simulink library "MIL_Test"  (Simulink 6.6)
undefined symbols (not defined in the file or in its folder): getdatatypespecs, slcm, StepSize
libraries: simulink x71, MIL_Test x6
(part 2 of 8)

== system MIL_Test/Test Data/Signal comparison/Range - Gap Absolute tolerance Precond ==
  Signal : Inport
  Reference : Inport  Port=2
  Abs : Abs
  Abs1 : Abs
  Absolute Tolerance : Constant  Value=AbsoluteTolerance
  Add : Sum  Inputs=+-  OutScaling=2^-10
  Relational Operator : RelationalOperator  Operator===  LogicOutDataTypeMode=Boolean
  Activate : Outport
  wires:
  Abs1/1 -> Relational Operator/2
  Absolute Tolerance/1 -> Abs1/1
  Reference/1 -> Add/2
  Signal/1 -> Add/1
  Add/1 -> Abs/1
  Abs/1 -> Relational Operator/1
  Relational Operator/1 -> Activate/1

== system MIL_Test/Test Data/Signal comparison/Range - Gap Relative tolerance Precond ==
  Signal : Inport
  Reference : Inport  Port=2
  Abs : Abs
  Abs1 : Abs
  Add : Sum  Inputs=+-  OutScaling=2^-10
  Divide1 : Product  Inputs=**/  OutScaling=2^-10
  Max : Constant  Value=100
  Relational Operator : RelationalOperator  Operator=<=  LogicOutDataTypeMode=Boolean
  Relative Tolerance : Constant
  Activate : Outport
  wires:
  Abs/1 -> Relational Operator/1
  Add/1 -> Abs/1
  Signal/1 -> Add/1
  Reference/1 -> Add/2, Abs1/1
  Divide1/1 -> Relational Operator/2
  Max/1 -> Divide1/3
  Relative Tolerance/1 -> Divide1/2
  Relational Operator/1 -> Activate/1
  Abs1/1 -> Divide1/1

== system MIL_Test/Test Data/Signal comparison/Range - Gap Tolerance range Precond ==
  Signal : Inport
  Lower bound : Inport  Port=2
  Upper bound : Inport  Port=3
  Logical Operator : Logic  AllPortsSameDT=off  OutDataTypeMode=Specify via dialog
  Relational Operator : RelationalOperator  LogicOutDataTypeMode=Boolean
  Relational Operator1 : RelationalOperator  LogicOutDataTypeMode=Boolean
  Activate : Outport
  wires:
  Upper bound/1 -> Relational Operator1/1
  Relational Operator/1 -> Logical Operator/2
  Relational Operator1/1 -> Logical Operator/1
  Signal/1 -> Relational Operator/1, Relational Operator1/2
  Logical Operator/1 -> Activate/1
  Lower bound/1 -> Relational Operator/2

== system MIL_Test/Test Data/Test Data Architecture/<Test data generator> ==
  Test Ctrl Influence : Inport
  Out Bus : Inport  Port=2
  <Requirement name> : Subsystem
  switch <signal1> : MultiPortSwitch  Inputs=1  zeroidx=on
  <signal1> : Outport
  wires:
  Test Ctrl Influence/1 -> switch <signal1>/1
  Out Bus/1 -> <Requirement name>/1(Out Bus)
  switch <signal1>/1 -> <signal1>/1
  <Requirement name>/1(<signal1>) -> switch <signal1>/2

== system MIL_Test/Test Quality/VFs Activation  Coverage/Max to date ==
  Signal : Inport
  Clock : Clock
      settings: Decimation=10
  Memory : Memory  Orientation=left
  MinMax : MinMax  Function=max  Inputs=2
  Switch : Switch  Criteria=u2 > Threshold
  Max : Outport
  wires:
  Memory/1 -> Switch/1
  Clock/1 -> Switch/2
  Switch/1 -> MinMax/1
  Signal/1 -> Switch/3, MinMax/2
  MinMax/1 -> Memory/1, Max/1

== system MIL_Test/Test Quality/VFs Activation  Coverage/Max to date1 ==
  Signal : Inport
  Clock : Clock
      settings: Decimation=10
  Memory : Memory  Orientation=left
  MinMax : MinMax  Function=max  Inputs=2
  Switch : Switch  Criteria=u2 > Threshold
  Max : Outport
  wires:
  Memory/1 -> Switch/1
  Clock/1 -> Switch/2
  Switch/1 -> MinMax/1
  Signal/1 -> Switch/3, MinMax/2
  MinMax/1 -> Memory/1, Max/1

== system MIL_Test/Validation Function/Feature extraction/Complete step detection ==
  Step : Inport
  Step response : Inport  Port=2
  Step detection : Subsystem  mask{MT=10, RT=0.001}
      mask prompts: MT "Minimal time for signals to be constant before a step"; RT "Relative tolerance for constant detection in %"
      mask CallbackString:
      | if (str2double(get_param(gcb,'MT')) < 0)
      |     error(['Minimal time specified (' get_param(gcb,'MT') ') negative. Please give a non-negative value.']);
      | else
      |     set_param([gcb '/Active if signals constant for some specified time/Min Time'],'Value',get_param(gcb,'MT'));
      | end|if or( (str2double(get_param(gcb,'RT')) < 0), (str2double(get_param(gcb,'RT')) > 100))
      |     error(['Relative tolerance value (' get_param(gcb,'RT') ') out of range. Please give a value between 0 and 100.']);
      | else
      |     set_param([gcb '/Active if signals constant for some specified time/Time since signal constant/Detect constant/Relative tolerance/Relative Tolerance'],'Value',get_param(gcb,'RT'));
      |     set_param([gcb '/Active if signals constant for some specified time/Time since signal constant/Detect constant'],'RT',get_param(gcb,'RT'));
      |     set_param([gcb '/Active if signals constant for some specified time/Time since signal constant'],'RT',get_param(gcb,'RT'));
      |     set_param([gcb '/Active if signals constant for some specified time/Time since signal constant1/Detect constant/Relative tolerance/Relative Tolerance'],'Value',get_param(gcb,'RT'));
      |     set_param([gcb '/Active if signals constant for some specified time/Time since signal constant1/Detect constant'],'RT',get_param(gcb,'RT'));
      |     set_param([gcb '/Active if signals constant for some specified time/Time since signal constant1'],'RT',get_param(gcb,'RT'));
      | end
  Step detection reset : Subsystem  mask{MT=10, RT=0.0001, MSS=10}
      mask prompts: MT "Minimal time for signals to be constant before a step"; RT "Relative tolerance for constant detection in %"; MSS "Minimal step size for step detection"
      mask CallbackString:
      | if (str2double(get_param(gcb,'MT')) < 0)
      |     error(['Minimal time specified (' get_param(gcb,'MT') ') negative. Please give a non-negative value.']);
      | else
      |     set_param([gcb '/Active if signals constant for some specified time/Min Time'],'Value',get_param(gcb,'MT'));
      | end|if or( (str2double(get_param(gcb,'RT')) < 0), (str2double(get_param(gcb,'RT')) > 100))
      |     error(['Relative tolerance value (' get_param(gcb,'RT') ') out of range. Please give a value between 0 and 100.']);
      | else
      |     set_param([gcb '/Active if signals constant for some specified time/Time since signal constant/Detect constant/Relative tolerance/Relative Tolerance'],'Value',get_param(gcb,'RT'));
      |     set_param([gcb '/Active if signals constant for some specified time/Time since signal constant/Detect constant'],'RT',get_param(gcb,'RT'));
      |     set_param([gcb '/Active if signals constant for some specified time/Time since signal constant'],'RT',get_param(gcb,'RT'));
      |     set_param([gcb '/Active if signals constant for some specified time/Time since signal constant1/Detect constant/Relative tolerance/Relative Tolerance'],'Value',get_param(gcb,'RT'));
      |     set_param([gcb '/Active if signals constant for some specified time/Time since signal constant1/Detect constant'],'RT',get_param(gcb,'RT'));
      |     set_param([gcb '/Active if signals constant for some specified time/Time since signal constant1'],'RT',get_param(gcb,'RT'));
      | end|if (str2double(get_param(gcb,'MSS')) < 0)
      |     error(['Minimal step size specified (' get_param(gcb,'MSS') ') negative. Please give a non-negative value.']);
      | else
      |     set_param([gcb '/Step detection/Min step size'],'Value',get_param(gcb,'MSS'));
      |     set_param([gcb '/Step detection'],'StepSize',get_param(gcb,'MSS'));
      | 
      | end
  R : Outport
  T : Outport  Port=2
  Complete step : Outport  Port=3
  wires:
  Step detection/1(End of complete step) -> T/1, Complete step/1
  Step detection reset/1(R) -> R/1, Step detection/1(R)
  Step response/1 -> Step detection reset/2(Step response), Step detection/3(Step response)
  Step/1 -> Step detection reset/1(Step), Step detection/2(Step)

== system MIL_Test/Validation Function/Feature extraction/Detect constant ==
  Signal : Inport
  Clock : Clock
      settings: Decimation=10
  Constant1 : Constant  Value=0  OutDataTypeMode=boolean
  Memory : Memory
  Relative tolerance : Subsystem
  Switch : Switch  Criteria=u2 > Threshold
  Constant : Outport
  wires:
  Switch/1 -> Constant/1
  Relative tolerance/1(sig == ref) -> Switch/1
  Clock/1 -> Switch/2
  Constant1/1 -> Switch/3
  Memory/1 -> Relative tolerance/2(ref)
  Signal/1 -> Relative tolerance/1(sig), Memory/1

== system MIL_Test/Validation Function/Feature extraction/Detect decrease ==
  Signal : Inport
  Clock : Clock
      settings: Decimation=10
  Memory : Memory
  Relational Operator : RelationalOperator  Operator=<  LogicOutDataTypeMode=Specify via dialog
  Switch : Switch  Criteria=u2 > Threshold
  Decrease : Outport
  wires:
  Signal/1 -> Relational Operator/1, Memory/1, Switch/3
  Relational Operator/1 -> Decrease/1
  Clock/1 -> Switch/2
  Memory/1 -> Switch/1
  Switch/1 -> Relational Operator/2

== system MIL_Test/Validation Function/Feature extraction/Detect increase ==
  Signal : Inport
  Clock : Clock
      settings: Decimation=10
  Memory : Memory
  Relational Operator : RelationalOperator  Operator=>  LogicOutDataTypeMode=Specify via dialog
  Switch : Switch  Criteria=u2 > Threshold
  Increase : Outport
  wires:
  Switch/1 -> Relational Operator/2
  Memory/1 -> Switch/1
  Clock/1 -> Switch/2
  Relational Operator/1 -> Increase/1
  Signal/1 -> Switch/3, Memory/1, Relational Operator/1

== system MIL_Test/Validation Function/Feature extraction/Linear relation ==
  y : Inport
  u : Inport  Port=2
  Product : Product  RndMeth=Zero
  Relative tolerance : Subsystem
  c : Constant  Value=5
  y == c u : Outport
  wires:
  Relative tolerance/1(sig == ref) -> y == c u/1
  c/1 -> Product/2
  u/1 -> Product/1
  Product/1 -> Relative tolerance/2(ref)
  y/1 -> Relative tolerance/1(sig)

== system MIL_Test/Validation Function/Feature extraction/Local maximum ==
  Signal : Inport
  Clock : Clock
      settings: Decimation=10
  Clock1 : Clock
      settings: Decimation=10
  Logical Operator : Logic  AllPortsSameDT=off  OutDataTypeMode=Boolean
  Memory : Memory
  Memory1 : Memory
  Relational Operator : RelationalOperator  Operator=<  LogicOutDataTypeMode=Boolean
  Relational Operator1 : RelationalOperator  Operator=>  LogicOutDataTypeMode=Boolean
  Switch : Switch  Criteria=u2 > Threshold
  Switch1 : Switch  Criteria=u2 > Threshold
  Maximum : Outport
  wires:
  Switch1/1 -> Relational Operator1/2
  Memory1/1 -> Switch1/1
  Clock1/1 -> Switch1/2
  Switch/1 -> Relational Operator1/1, Switch1/3, Memory1/1, Relational Operator/2
  Memory/1 -> Switch/1
  Clock/1 -> Switch/2
  Relational Operator/1 -> Logical Operator/1
  Relational Operator1/1 -> Logical Operator/2
  Logical Operator/1 -> Maximum/1
  Signal/1 -> Switch/3, Memory/1, Relational Operator/1

== system MIL_Test/Validation Function/Feature extraction/Min to date ==
  Signal : Inport
  Clock : Clock
      settings: Decimation=10
  Memory : Memory  Orientation=left
  MinMax : MinMax  Inputs=2
  Switch : Switch  Criteria=u2 > Threshold
  Min : Outport
  wires:
  Memory/1 -> Switch/1
  Clock/1 -> Switch/2
  Switch/1 -> MinMax/1
  Signal/1 -> Switch/3, MinMax/2
  MinMax/1 -> Memory/1, Min/1

== system MIL_Test/Validation Function/Feature extraction/Moving average ==
  Signal : Inport
  Add : Sum  OutScaling=2^-10
  Clock : Clock
      settings: Decimation=10
  Constant : Constant  Value=2
  Divide : Product  Inputs=*/  OutScaling=2^-10
  Memory : Memory
  Switch : Switch  Criteria=u2 > Threshold
  MA : Outport
  wires:
  Switch/1 -> Add/2
  Memory/1 -> Switch/1
  Clock/1 -> Switch/2
  Signal/1 -> Add/1, Switch/3, Memory/1
  Add/1 -> Divide/1
  Constant/1 -> Divide/2
  Divide/1 -> MA/1

== system MIL_Test/Validation Function/Feature extraction/Peak detection ==
  Signal : Inport
  Abs : Abs
  Abs1 : Abs
  Add : Sum  Inputs=+-  OutScaling=2^-10
  Add1 : Sum  Inputs=+-  OutScaling=2^-10
  Clock : Clock
      settings: Decimation=10
  Clock1 : Clock
      settings: Decimation=10
  Compare To Zero : simulink/Logic and Bit Operations/Compare To Zero  SystemSampleTime=-1  relop=<=  LogicOutDataTypeMode=boolean  ZeroCross=off
  Logical Operator : Logic  Inputs=3  AllPortsSameDT=off  OutDataTypeMode=Boolean
  Memory : Memory
  Memory1 : Memory
  Product : Product  RndMeth=Zero
  Relational Operator : RelationalOperator  Operator=<=  LogicOutDataTypeMode=Boolean
  Relational Operator1 : RelationalOperator  LogicOutDataTypeMode=Boolean
  Sensibility1 : Constant  Value=0.198
  Sensibility2 : Constant  Value=0.198
  Switch : Switch  Criteria=u2 > Threshold
  Switch1 : Switch  Criteria=u2 > Threshold
  Peak : Outport
  wires:
  Sensibility2/1 -> Relational Operator1/2
  Abs1/1 -> Relational Operator1/1
  Sensibility1/1 -> Relational Operator/1
  Abs/1 -> Relational Operator/2
  Product/1 -> Compare To Zero/1
  Compare To Zero/1 -> Logical Operator/2
  Relational Operator1/1 -> Logical Operator/3
  Relational Operator/1 -> Logical Operator/1
  Add1/1 -> Product/2, Abs1/1
  Signal/1 -> Memory/1, Switch/3, Add/1
  Logical Operator/1 -> Peak/1
  Clock/1 -> Switch/2
  Memory/1 -> Switch/1
  Switch/1 -> Add1/1, Add/2, Memory1/1, Switch1/3
  Clock1/1 -> Switch1/2
  Memory1/1 -> Switch1/1
  Switch1/1 -> Add1/2
  Add/1 -> Product/1, Abs/1

== system MIL_Test/Validation Function/Feature extraction/Signal value @ maximum ==
  Signal : Inport
  Local maximum : Subsystem  TreatAsAtomicUnit=on
  Trigger : Outport
  Feature : Outport  Port=2
  wires:
  Local maximum/1(Maximum) -> Trigger/1
  Signal/1 -> Local maximum/1(Signal), Feature/1

== system MIL_Test/Validation Function/Feature extraction/Step detection ==
  Signal : Inport
  Abs : Abs
  Add : Sum  Inputs=+-  OutScaling=2^-10
  Clock : Clock
      settings: Decimation=10
  Memory : Memory
  Min step size : Constant
  Relational Operator : RelationalOperator  LogicOutDataTypeMode=Boolean
  Switch : Switch  Criteria=u2 > Threshold
  Step : Outport
  wires:
  Switch/1 -> Add/2
  Memory/1 -> Switch/1
  Clock/1 -> Switch/2
  Signal/1 -> Add/1, Switch/3, Memory/1
  Abs/1 -> Relational Operator/1
  Min step size/1 -> Relational Operator/2
  Relational Operator/1 -> Step/1
  Add/1 -> Abs/1

== system MIL_Test/Validation Function/Feature extraction/Step response characteristics ==
  Step : Inport
  Step response : Inport  Port=2
  Step response characteristics extraction : Subsystem  mask(Step response feature extraction){gain=0.8333, lowerLim=10, upperLim=90, MOma=ones(1,10), RelTol=0.1, MinTime=1, Range=5, sseW=ones(1,10)}
      mask prompts: gain "System's static gain"; lowerLim "Rise time interval lower limit (in set point %)"; upperLim "Rise time interval upper limit (in set point %)"; MOma "Maximum overshoot moving average weights"; RelTol "Maximum overshoot - Detect constant if no overshoot - Relative Tolerance"; MinTime "Maximum overshoot - Detect constant if no overshoot - Minimum constant time"; Range "Settling time range (in set point %)"; sseW "Steady state error - moving average weights"
      mask help: Extracts four step response feature characteristics. Extraction parameters are shown below.
      mask CallbackString:
      | set_param([gcb '/Static Gain'],'Value',get_param(gcb,'gain'));|set_param([gcb '/Extract rise time/lowerLim'],'Value',get_param(gcb,'lowerLim'));|set_param([gcb '/Extract rise time/upperLim'],'Value',get_param(gcb,'upperLim'));|set_param([gcb '/Extract maximum overshoot/Step response moving average and initial conditions before step/Weighted Moving Average'],'mgainval',get_param(gcb,'MOma'));
      | set_param([gcb '/Extract maximum overshoot/Step response moving average and initial conditions before step/Weighted Moving Average1'],'mgainval',get_param(gcb,'MOma'));|set_param([gcb '/Extract maximum overshoot/Active if signals constant for some specified time/Time since signal constant'],'RT',get_param(gcb,'RelTol'));
      | set_param([gcb '/Extract maximum overshoot/Active if signals constant for some specified time/Time since signal constant1'],'RT',get_param(gcb,'RelTol'));|set_param([gcb '/Extract maximum overshoot/Active if signals constant for some specified time/Min Time'],'Value',get_param(gcb,'MinTime'));|set_param([gcb '/Extract settling time/Set point percent'],'Value',get_param(gcb,'Range'));|set_param([gcb '/Extract steady state error/Weighted Moving Average'],'mgainval',get_param(gcb,'sseW'));
  Step response reset : Subsystem  mask{MT=1, RT=0.0001, MSS=1}
      mask prompts: MT "Minimal time for signals to be constant before a step"; RT "Relative tolerance for constant detection in %"; MSS "Minimal step size for step detection"
      mask CallbackString:
      | if (str2double(get_param(gcb,'MT')) < 0)
      |     error(['Minimal time specified (' get_param(gcb,'MT') ') negative. Please give a non-negative value.']);
      | else
      |     set_param([gcb '/Active if signals constant for some specified time/Min Time'],'Value',get_param(gcb,'MT'));
      | end|if or( (str2double(get_param(gcb,'RT')) < 0), (str2double(get_param(gcb,'RT')) > 100))
      |     error(['Relative tolerance value (' get_param(gcb,'RT') ') out of range. Please give a value between 0 and 100.']);
      | else
      |     set_param([gcb '/Active if signals constant for some specified time/Time since signal constant/Detect constant/Relative tolerance/Relative Tolerance'],'Value',get_param(gcb,'RT'));
      |     set_param([gcb '/Active if signals constant for some specified time/Time since signal constant/Detect constant'],'RT',get_param(gcb,'RT'));
      |     set_param([gcb '/Active if signals constant for some specified time/Time since signal constant'],'RT',get_param(gcb,'RT'));
      |     set_param([gcb '/Active if signals constant for some specified time/Time since signal constant1/Detect constant/Relative tolerance/Relative Tolerance'],'Value',get_param(gcb,'RT'));
      |     set_param([gcb '/Active if signals constant for some specified time/Time since signal constant1/Detect constant'],'RT',get_param(gcb,'RT'));
      |     set_param([gcb '/Active if signals constant for some specified time/Time since signal constant1'],'RT',get_param(gcb,'RT'));
      | end|if (str2double(get_param(gcb,'MSS')) < 0)
      |     error(['Minimal step size specified (' get_param(gcb,'MSS') ') negative. Please give a non-negative value.']);
      | else
      |     set_param([gcb '/Step detection/Min step size'],'Value',get_param(gcb,'MSS'));
      |     set_param([gcb '/Step detection'],'StepSize',get_param(gcb,'MSS'));
      | 
      | end
  Step response trigger : Subsystem  mask(Step response trigger extraction){MinTime=1, RelTol=0.5, MAXsse=0.5}
      mask prompts: MinTime "Detect constant signals - Minimum constant time"; RelTol "Detect constant signals - Relative Tolerance"; MAXsse "Maximum steady state error for triggering"
      mask help: This block extracts the trigger signals for the four step response characteristics.
      mask CallbackString:
      | set_param([gcb '/Active if signals constant for some specified time/Min Time'],'Value',get_param(gcb,'MinTime'));|set_param([gcb '/Active if signals constant for some specified time/Time since signal constant'],'RT',get_param(gcb,'RelTol'));
      | set_param([gcb '/Active if signals constant for some specified time/Time since signal constant1'],'RT',get_param(gcb,'RelTol'));|set_param([gcb '/Compare To Constant'],'const',get_param(gcb,'MAXsse'));
  R : Outport
  Rise time T : Outport  Port=2  DataType=double
  Overshoot T : Outport  Port=3  DataType=double
  Settling time T : Outport  Port=4  DataType=double
  Steady state error T : Outport  Port=5  DataType=double
  Rise time : Outport  Port=6
  Maximum Overshoot : Outport  Port=7
  Settling time : Outport  Port=8  DataType=double
  Steady state error : Outport  Port=9  DataType=double
  wires:
  Step response trigger/4(Steady state error T) -> Steady state error T/1
  Step response trigger/3(Settling time T) -> Settling time T/1
  Step response trigger/2(Overshoot T) -> Overshoot T/1
  Step response trigger/1(Rise time T) -> Rise time T/1
  Step response characteristics extraction/2(Maximum overshoot) -> Maximum Overshoot/1
  Step response characteristics extraction/3(Settling time) -> Settling time/1
  Step response characteristics extraction/1(Rise time) -> Rise time/1
  Step response/1 -> Step response trigger/2(Step response), Step response characteristics extraction/3(Step response), Step response reset/2(Step response)
  Step/1 -> Step response characteristics extraction/2(Step), Step response reset/1(Step)
  Step response characteristics extraction/4(Steady state error) -> Steady state error/1, Step response trigger/1(Steady state error)
  Step response reset/1(R) -> Step response characteristics extraction/1(R), R/1

== system MIL_Test/Validation Function/Feature extraction/Time @ sig = x ==
  Signal : Inport
  Clock : Clock
      settings: Decimation=10
  Relative tolerance : Subsystem
  Trigger Value : Constant  Value=5
  Trigger : Outport
  Feature : Outport  Port=2
  wires:
  Clock/1 -> Feature/1
  Trigger Value/1 -> Relative tolerance/2(ref)
  Signal/1 -> Relative tolerance/1(sig)
  Relative tolerance/1(sig == ref) -> Trigger/1

== system MIL_Test/Validation Function/Feature extraction/Time since signal constant ==
  Signal : Inport
  Clock : Clock
      settings: Decimation=10
  Detect constant : Subsystem  TreatAsAtomicUnit=on  mask(Feature extraction block){RT=1}
      mask prompts: RT "Relative tolerance in %"
      mask help: Detect if the signal value is constant (using the last two signal values) allowing for a user-defined relative deviation
      mask CallbackString:
      | if or( (str2double(get_param(gcb,'RT')) < 0), (str2double(get_param(gcb,'RT')) > 100))
      |     error(['Relative tolerance value (' get_param(gcb,'RT') ') out of range. Please give a value between 0 and 100.']);
      | else
      |     set_param([gcb '/Relative tolerance/Relative Tolerance'],'Value',get_param(gcb,'RT'));
      | end
  Logical Operator : Logic  Operator=NAND  AllPortsSameDT=off  OutDataTypeMode=Boolean
  Logical Operator1 : Logic  Operator=NOT  AllPortsSameDT=off  OutDataTypeMode=Boolean
  Memory : Memory  Orientation=left
  Memory1 : Memory
  Subtract : Sum  Inputs=-+  OutScaling=2^-10
  Switch : Switch  Criteria=u2 > Threshold
  Trigger : Outport
  Feature : Outport  Port=2
  wires:
  Logical Operator/1 -> Switch/2
  Logical Operator1/1 -> Logical Operator/2
  Memory1/1 -> Logical Operator1/1
  Memory/1 -> Switch/1
  Switch/1 -> Memory/1, Subtract/1
  Clock/1 -> Switch/3, Subtract/2
  Subtract/1 -> Feature/1
  Detect constant/1(Constant) -> Memory1/1, Logical Operator/1, Trigger/1
  Signal/1 -> Detect constant/1(Signal)

== system MIL_Test/Validation Function/Signal comparison/Bound Ass ==
  Signal : Inport
  Reference : Inport  Port=2
  Bus Creator : BusCreator  Inputs=5
  Data Type Conversion{,1..3} (4 alike) : DataTypeConversion
  Delay : Constant  Value=0
  LOWER : Constant  Value=Lower  OutDataTypeMode=int8
  No Limit : Constant  Value=Inf
  No limit : Constant  Value=-Inf
  Relational Operator : RelationalOperator  Operator=<=  LogicOutDataTypeMode=Boolean  LogicDataType=double
  Switch 2 : Switch  Criteria=u2 ~= 0
  Switch 3 : Switch  Criteria=u2 ~= 0
  UPPER : Constant  Value=Upper  OutDataTypeMode=int8
  V : Outport  InitialOutput=[2]
  wires:
  Relational Operator/1 -> Data Type Conversion/1
  Data Type Conversion3/1 -> Bus Creator/4  "Actual data"
  Data Type Conversion2/1 -> Bus Creator/3  "Expected upper limit"
  Data Type Conversion1/1 -> Bus Creator/2  "Expected lower limit"
  Data Type Conversion/1 -> Bus Creator/1  "Local verdict"
  Bus Creator/1 -> V/1
  Reference/1 -> Relational Operator/2, Switch 2/3, Switch 3/3
  Signal/1 -> Data Type Conversion3/1, Relational Operator/1
  UPPER/1 -> Switch 3/2
  No Limit/1 -> Switch 3/1
  LOWER/1 -> Switch 2/2
  No limit/1 -> Switch 2/1
  Switch 2/1 -> Data Type Conversion1/1
  Switch 3/1 -> Data Type Conversion2/1
  Delay/1 -> Bus Creator/5  "Delay"

== system MIL_Test/Validation Function/Signal comparison/Bound Precond ==
  Signal : Inport
  Reference : Inport  Port=2
  RelOp : RelationalOperator  LogicOutDataTypeMode=Specify via dialog
  Activate : Outport
  wires:
  Signal/1 -> RelOp/1
  RelOp/1 -> Activate/1
  Reference/1 -> RelOp/2

== system MIL_Test/Validation Function/Signal comparison/Range - Gap Absolute tolerance Ass ==
  Signal : Inport
  Reference : Inport  Port=2
  Abs : Abs
  Abs1 : Abs
  Absolute Tolerance : Constant  Value=AbsoluteTolerance
  Add : Sum  Inputs=+-  OutScaling=2^-10
  Add1 : Sum  Inputs=+-  OutScaling=2^-10
  Add2 : Sum  OutScaling=2^-10
  Bus Creator : BusCreator  Inputs=5
  Data Type Conversion{,1..3} (4 alike) : DataTypeConversion
  Delay : Constant  Value=0
  Relational Operator : RelationalOperator  Operator===  LogicOutDataTypeMode=Boolean
  V : Outport  InitialOutput=[2]
  wires:
  Abs1/1 -> Relational Operator/2, Add2/2, Add1/2
  Absolute Tolerance/1 -> Abs1/1
  Reference/1 -> Add/2, Add2/1, Add1/1
  Signal/1 -> Add/1, Data Type Conversion3/1
  Add/1 -> Abs/1
  Abs/1 -> Relational Operator/1
  Relational Operator/1 -> Data Type Conversion/1
  Delay/1 -> Bus Creator/5  "Delay"
  Add2/1 -> Data Type Conversion2/1
  Add1/1 -> Data Type Conversion1/1
  Bus Creator/1 -> V/1
  Data Type Conversion/1 -> Bus Creator/1  "Local verdict"
  Data Type Conversion1/1 -> Bus Creator/2  "Expected lower limit"
  Data Type Conversion2/1 -> Bus Creator/3  "Expected upper limit"
  Data Type Conversion3/1 -> Bus Creator/4  "Actual data"

== system MIL_Test/Validation Function/Signal comparison/Range - Gap Absolute tolerance Precond ==
  Signal : Inport
  Reference : Inport  Port=2
  Abs : Abs
  Abs1 : Abs
  Absolute Tolerance : Constant  Value=AbsoluteTolerance
  Add : Sum  Inputs=+-  OutScaling=2^-10
  Relational Operator : RelationalOperator  Operator===  LogicOutDataTypeMode=Boolean
  Activate : Outport
  wires:
  Relational Operator/1 -> Activate/1
  Abs/1 -> Relational Operator/1
  Add/1 -> Abs/1
  Signal/1 -> Add/1
  Reference/1 -> Add/2
  Absolute Tolerance/1 -> Abs1/1
  Abs1/1 -> Relational Operator/2

== system MIL_Test/Validation Function/Signal comparison/Range - Gap Relative tolerance Ass ==
  Signal : Inport
  Reference : Inport  Port=2
  Abs : Abs
  Abs1 : Abs
  Add : Sum  Inputs=+-  OutScaling=2^-10
  Add1 : Sum  Inputs=+-  OutScaling=2^-10
  Add2 : Sum  OutScaling=2^-10
  Bus Creator : BusCreator  Inputs=5
  Data Type Conversion{,1..3} (4 alike) : DataTypeConversion
  Delay : Constant  Value=0
  Divide1 : Product  Inputs=**/  OutScaling=2^-10
  Max : Constant  Value=100
  Relational Operator : RelationalOperator  Operator=<=  LogicOutDataTypeMode=Boolean
  Relative Tolerance : Constant
  V : Outport  InitialOutput=[2]
  wires:
  Abs/1 -> Relational Operator/1
  Add/1 -> Abs/1
  Signal/1 -> Add/1, Data Type Conversion3/1
  Reference/1 -> Add/2, Abs1/1, Add2/2, Add1/1
  Divide1/1 -> Relational Operator/2, Add1/2, Add2/1
  Max/1 -> Divide1/3
  Relative Tolerance/1 -> Divide1/2
  Relational Operator/1 -> Data Type Conversion/1
  Abs1/1 -> Divide1/1
  Delay/1 -> Bus Creator/5  "Delay"
  Add2/1 -> Data Type Conversion2/1
  Add1/1 -> Data Type Conversion1/1
  Bus Creator/1 -> V/1
  Data Type Conversion/1 -> Bus Creator/1  "Local verdict"
  Data Type Conversion1/1 -> Bus Creator/2  "Expected lower limit"
  Data Type Conversion2/1 -> Bus Creator/3  "Expected upper limit"
  Data Type Conversion3/1 -> Bus Creator/4  "Actual data"

== system MIL_Test/Validation Function/Signal comparison/Range - Gap Relative tolerance Precond ==
  Signal : Inport
  Reference : Inport  Port=2
  Abs : Abs
  Abs1 : Abs
  Add : Sum  Inputs=+-  OutScaling=2^-10
  Divide1 : Product  Inputs=**/  OutScaling=2^-10
  Max : Constant  Value=100
  Relational Operator : RelationalOperator  Operator=<=  LogicOutDataTypeMode=Boolean
  Relative Tolerance : Constant
  Activate : Outport
  wires:
  Abs1/1 -> Divide1/1
  Relational Operator/1 -> Activate/1
  Relative Tolerance/1 -> Divide1/2
  Max/1 -> Divide1/3
  Divide1/1 -> Relational Operator/2
  Reference/1 -> Abs1/1, Add/2
  Signal/1 -> Add/1
  Add/1 -> Abs/1
  Abs/1 -> Relational Operator/1

== system MIL_Test/Validation Function/Signal comparison/Range - Gap Tolerance range Ass ==
  Signal : Inport
  Lower bound : Inport  Port=2
  Upper bound : Inport  Port=3
  Bus Creator : BusCreator  Inputs=5
  Data Type Conversion{,1..3} (4 alike) : DataTypeConversion
  Delay : Constant  Value=0
  Logical Operator : Logic  AllPortsSameDT=off  OutDataTypeMode=Specify via dialog
  Relational Operator : RelationalOperator  LogicOutDataTypeMode=Boolean
  Relational Operator1 : RelationalOperator  LogicOutDataTypeMode=Boolean
  V : Outport  InitialOutput=[2]
  wires:
  Upper bound/1 -> Relational Operator1/1, Data Type Conversion2/1
  Relational Operator/1 -> Logical Operator/2
  Relational Operator1/1 -> Logical Operator/1
  Signal/1 -> Relational Operator/1, Relational Operator1/2, Data Type Conversion3/1
  Logical Operator/1 -> Data Type Conversion/1
  Lower bound/1 -> Relational Operator/2, Data Type Conversion1/1
  Delay/1 -> Bus Creator/5  "Delay"
  Bus Creator/1 -> V/1
  Data Type Conversion/1 -> Bus Creator/1  "Local verdict"
  Data Type Conversion1/1 -> Bus Creator/2  "Expected lower limit"
  Data Type Conversion2/1 -> Bus Creator/3  "Expected upper limit"
  Data Type Conversion3/1 -> Bus Creator/4  "Actual data"

== system MIL_Test/Validation Function/Signal comparison/Range - Gap Tolerance range Precond ==
  Signal : Inport
  Lower bound : Inport  Port=2
  Upper bound : Inport  Port=3
  Logical Operator : Logic  AllPortsSameDT=off  OutDataTypeMode=Specify via dialog
  Relational Operator : RelationalOperator  LogicOutDataTypeMode=Boolean
  Relational Operator1 : RelationalOperator  LogicOutDataTypeMode=Boolean
  Activate : Outport
  wires:
  Lower bound/1 -> Relational Operator/2
  Logical Operator/1 -> Activate/1
  Signal/1 -> Relational Operator1/2, Relational Operator/1
  Relational Operator1/1 -> Logical Operator/1
  Relational Operator/1 -> Logical Operator/2
  Upper bound/1 -> Relational Operator1/1

== system MIL_Test/Validation Function/TODO/<system name> ==
  InOut Bus : Inport
  <Requirement name> : Subsystem  Description=Requirement template. Create a new requirement from this template.
  Bus Creator : BusCreator  Inputs=1
  Signal Conversion : SignalConversion  ConversionOutput=Bus copy
  Terminator : Terminator
  wires:
  InOut Bus/1 -> Signal Conversion/1
  Bus Creator/1 -> Terminator/1
  <Requirement name>/1(Test Info) -> Bus Creator/1
  Signal Conversion/1 -> <Requirement name>/1(InOut Bus)

== system MIL_Test/Validation Function/TODO/Assertions ==
  Activate : Inport
  InOut Bus : Inport  Port=2
  Fault info : Subsystem  TreatAsAtomicUnit=on  mask{Ass=[65   99   99   80  101  100   97  108   32   61   61   32   49], Pre=[73  110   79  117  116   10   66  117  115], Req=[83   82   45   80   73   45   48   49   46   51   10   65   99   99  101  108  101  114   97  116  105  111  110   10   80  101  100   97  108   32  114  101   99  111  103  110  105  116  105  111  110]}
      mask prompts: Req "Mask Parameter 3:"
      mask init:
      | set_param(gcb, ...
      |           'Ass', ...
      |           ['[' num2str(uint8(get_param(get_param(gcb,'Parent'),'Name'))) ']']);
      | LinesToAss = getfield(get_param(get_param(get_param(gcb,'Parent'),'handle'),'LineHandles'),'Inport');
      | LinePreToAss = LinesToAss(1);
      | set_param(gcb, ...
      |           'Pre', ...
      |           ['[' num2str(uint8(get_param(get_param(LinePreToAss,'SrcBlockHandle'),'Name'))) ']']); 
      | set_param(gcb, ...
      |           'Req', ...
      |           ['[' num2str(uint8(get_param(get_param(get_param(get_param(gcb,'Parent'),'handle'),'Parent'),'Name'))) ']']);
      | clear LinesToAss LinePreToAss;
  Signal comparison : Subsystem
  VF info : Outport

== system MIL_Test/Validation Function/TODO/Model Info ==
  EmptySubsystem : Subsystem

== system MIL_Test/Validation Function/TODO/Preconditions ==
  Signal comparison : Subsystem

== system MIL_Test/Validation Function/TODO/TD determinate (TD D) ==
  Signal : Inport
  Trigger : Outport
  Feature : Outport  Port=2

== system MIL_Test/Validation Function/TODO/TD immediate (TD I) ==
  Signal : Inport
  Trigger : Outport
  Feature : Outport  Port=2

== system MIL_Test/Validation Function/TODO/TD indeterminate ==
  Signal : Inport
  R : Outport
  T : Outport  Port=2
  Feature : Outport  Port=3

== system MIL_Test/Validation Function/TODO/TD indeterminate, limited (TD IL) ==
  Signal : Inport
  R : Outport
  T : Outport  Port=2
  Feature : Outport  Port=3

== system MIL_Test/Validation Function/TODO/TI determinate (TI D) ==
  Signal : Inport
  Feature : Outport

== system MIL_Test/Validation Function/TODO/TI immediate (TI I) ==
  Signal : Inport
  Feature : Outport

== system MIL_Test/Validation Function/TODO/Validation FunctionsTemplate ==
  InOut Bus : Inport
  Arbitration : Subsystem
  Bus Creator : BusCreator  Inputs=2
  Bus Creator4 : BusCreator  Inputs=2
  Bus Selector : BusSelector  OutputSignals=signal1.signal1
  Datatype conversion : Subsystem  TreatAsAtomicUnit=on
  Requirement : Subsystem  mask{No=1}
      mask prompts: No "Number of single Validation Functions"
      mask StyleString: popup(1|2|3|4|5|6|7|8|9|10|11|12|13|14|15|16|17|18|19|20)
      mask CallbackString: ReqInVF_callback(gcb);
  Requirement2 : Subsystem  mask{No=1}
      mask prompts: No "Number of single Validation Functions"
      mask StyleString: popup(1|2|3|4|5|6|7|8|9|10|11|12|13|14|15|16|17|18|19|20)
      mask CallbackString: ReqInVF_callback(gcb);
  Terminator : Terminator
  ReqVerdict Bus : Outport
  Overall Verdict : Outport  Port=2
  wires:
  Bus Selector/1 -> Arbitration/1(In1), Bus Creator4/1  "<signal1>"
  Bus Creator4/1 -> ReqVerdict Bus/1
  Datatype conversion/1(InOut Bus) -> Requirement/1(InOut Bus), Requirement2/1(InOut Bus)
  Arbitration/1(Out1) -> Overall Verdict/1
  Requirement/1(Validation Information) -> Bus Creator/1
  Bus Creator/1 -> Terminator/1, Bus Selector/1
  InOut Bus/1 -> Datatype conversion/1(InOutBus)
  Requirement2/1(Validation Information) -> Bus Creator/2

== system MIL_Test/Validation Function/Test Evaluation Architecture/<system name> ==
  InOut  Bus : Inport
  <Requirement name> : Subsystem  Description=Requirement template. Create a new requirement from this template.  mask{No=1}
      mask prompts: No "Number of single Validation Functions"
      mask StyleString: popup(1|2|3|4|5|6|7|8|9|10|11|12|13|14|15|16|17|18|19|20)
      mask CallbackString: ReqName_callback(gcb);
  Arbitration : Subsystem
  Bus Creator : BusCreator  Inputs=1
  Bus Creator1 : BusCreator  Inputs=2
  Bus Creator4 : BusCreator  Inputs=1
  Bus Selector : BusSelector  OutputSignals=signal1.signal1.signal1
  Signal Conversion : SignalConversion  ConversionOutput=Bus copy
  Terminator : Terminator
  Eval Results : Outport
  wires:
  Bus Selector/1 -> Bus Creator4/1, Arbitration/1(In1)  "<signal1>"
  Arbitration/1(Out1) -> Bus Creator1/1
  <Requirement name>/1(Test Info) -> Bus Creator/1
  InOut  Bus/1 -> Signal Conversion/1
  Bus Creator/1 -> Bus Selector/1, Terminator/1
  Signal Conversion/1 -> <Requirement name>/1(InOut Bus)
  Bus Creator4/1 -> Bus Creator1/2
  Bus Creator1/1 -> Eval Results/1

== system MIL_Test/Validation Function/Test Evaluation Architecture/Alternative ==
  InOut Bus : Inport
  Alternative Arbitration : Stateflow chart
  Assertions : MIL_Test/Validation Function/Validation FunctionsTemplate/Requirement/Assertions
  Assertions1 : MIL_Test/Validation Function/Validation FunctionsTemplate/Requirement/Assertions
  Assertions2 : MIL_Test/Validation Function/Validation FunctionsTemplate/Requirement/Assertions
  Preconditions : MIL_Test/Validation Function/Validation FunctionsTemplate/Requirement/Preconditions
  Alternative OverallVerdict : Outport
  wires:
  Preconditions/1 -> Assertions/1, Assertions1/1, Assertions2/1
  InOut Bus/1 -> Preconditions/1, Assertions/2, Assertions1/2, Assertions2/2
  Assertions/1 -> Alternative Arbitration/1(LocalVerdict1)
  Assertions1/1 -> Alternative Arbitration/2(LocalVerdict2)
  Assertions2/1 -> Alternative Arbitration/3(LocalVerdict3)
  Alternative Arbitration/1(OverallVerdict) -> Alternative OverallVerdict/1

== system MIL_Test/Test Control/Test Control Architecture/Connection Helpers/TestControl for  TestCases Sequencing ==

== system MIL_Test/Test Control/Test Control Architecture/Connection Helpers/TestControl for  TestCases Sequencing NoMask ==
  @StopTime1 : Inport
  @[t1,t2]1 : Inport  Port=2
  @Time1 : Inport  Port=3
  FulfillmentAtTime 2 : ToWorkspace  VariableName=FulfillmentAtTime1  SampleTime=-1  SaveFormat=Structure With Time
  FulfillmentAtTime1 : Display
  FulfillmentDuring 1 : ToWorkspace  VariableName=FulfillmentDuring1  SampleTime=-1  SaveFormat=Structure With Time
  FulfillmentDuring1 : Display
  FulfillmentStopTime 1 : ToWorkspace  VariableName=FulfillmentStopTime1  SampleTime=-1  SaveFormat=Structure With Time
  FulfillmentStopTime1 : Display
  IF Signal@SimStopTime for TC = value1 : Subsystem  mask(Check if Incoming Signal has an Expected Value @ Simulation Stop Time){currentStopTime=on, condition=0}
      mask prompts: currentStopTime "Check @ End of Simulation"; condition "Signal should equal to"
      mask help:
      | The Subsystem checks if the incoming signal (i.e. Overall Verdict, single Requirement Local Verdict, or SUT Outputs) has an expected value at the end of simulation of a previously specified testcase.
      | ____________________________________________________________________
      | 'Check @ End of Simulation' gets the simulation stop time from the window in Simulink.
      | 'Signal should equal to:' is used for giving the condition for the value of signal (i.e.):
      | 2 = none
      | 1 = pass
      | 0 = fail
      | X = anyNumber
      | The subsystem outputs 1 if the condition is fullfilled.
      mask init:
      | % p=get_param(gcb, 'PortHandles');
      | % l=get_param(p.Inport, 'Line'); 
      | % Inp=get_param(p.Inport, 'Name');
      | % set_param(Inp, 'Name', get_param(l, 'Name'));
      mask CallbackString:
      | block = gcb;
      | TCtblock = get_param(get_param(block, 'Parent'), 'Parent');
      | currentStopTime = get_param(TCtblock, 'StopTime');|
  "IF signal @[timeUp, timeDown] for TC = value1" : Subsystem  mask(Check if Incoming Signal has an Expected Value in the given Period of Time){timeDown=11, timeUp=155, condition=1}
      mask prompts: timeDown "Check @ Time from:"; timeUp "Check @ Time till:"; condition "Signal should equal to:"
      mask help:
      | The Subsystem checks if the incoming signal (i.e. Overall Verdict, single Requirement Local Verdict, or SUT Outputs) has an expected value in the given period of time of a previously specified testcase.
      | ____________________________________________________________________
      | 'Check @ Time from:' means the time where the check should begin.
      | 'Check @ Time till:' means the time where the check should end.
      | Constraint: TimeUp > TimeDown.
      | 'Signal should equal to:' is used for giving the condition for the value of signal (i.e.):
      | 2 = none
      | 1 = pass
      | 0 = fail
      | X = anyNumber
      | The subsystem outputs 1 if the condition is fullfilled.
      mask init:
      | % p=get_param(gcb, 'PortHandles');
      | % l=get_param(p.Inport, 'Line'); 
      | % Inp=get_param(p.Inport, 'Name');
      | % set_param(Inp, 'Name', get_param(l, 'Name'));
      mask CallbackString: timeDown = str2double(get_param(gcb,'timeDown'));|timeUp = str2double(get_param(gcb,'timeUp'));|
  IF signal@time for TC = value1 : Subsystem  mask(Check if Incoming Signal has an Expected Value @ given Time){time=22, condition=1}
      mask prompts: time "Check @ Time t"; condition "Signal should equal to"
      mask help:
      | The Subsystem checks if the incoming signal (i.e. Overall Verdict, single Requirement Local Verdict, or SUT Outputs) has an expected value at given time of a previously specified testcase.
      | ____________________________________________________________________
      | 'Check @ Time t' means the time point when the condition should be checked.
      | 'Signal should equal to:' is used for giving the condition for the value of signal (i.e.):
      | 2 = none
      | 1 = pass
      | 0 = fail
      | X = anyNumber
      | The subsystem outputs 1 if the condition is fullfilled.
      mask CallbackString: time = str2double(get_param(gcb,'time'));|
  wires:
  IF signal@time for TC = value1/1(Fulfillment) -> FulfillmentAtTime 2/1, FulfillmentAtTime1/1
  @Time1/1 -> IF signal@time for TC = value1/1(Signal)
  "IF signal @[timeUp, timeDown] for TC = value1"/1(Fulfillment) -> FulfillmentDuring 1/1, FulfillmentDuring1/1
  @[t1,t2]1/1 -> "IF signal @[timeUp, timeDown] for TC = value1"/1(Signal)
  IF Signal@SimStopTime for TC = value1/1(Fulfillment) -> FulfillmentStopTime 1/1, FulfillmentStopTime1/1
  @StopTime1/1 -> IF Signal@SimStopTime for TC = value1/1(Signal)

== system MIL_Test/Test Control/Test Control Architecture/Connection Helpers/TestControl for  TestCases SequencingTemplate ==

== system MIL_Test/Test Control/Test Control Architecture/Test Control  depending on Verdict/Counter ==
  In1 : Inport
  Trigger : TriggerPort
  " 1" : DataTypeConversion  Orientation=down
  Add : Sum  OutScaling=2^-10
  Memory : Memory  Orientation=left  InheritSampleTime=on
  Number of triggers : Constant  Value=2
  Relational Operator1 : RelationalOperator  Operator===  LogicOutDataTypeMode=Boolean
  Scope1 : Scope  NumInputPorts=4
      settings: YMin=182.932~-5~-5~-5  YMax=202.188~5~5~5  SaveName=ScopeData14  MaxDataPoints=5000000
  Out1 : Outport
  wires:
  In1/1 -> Add/1, Scope1/2
  Number of triggers/1 -> Relational Operator1/2
  Relational Operator1/1 -> Out1/1
  Add/1 -> " 1"/1, Relational Operator1/1, Scope1/3
  Memory/1 -> Add/2
  " 1"/1 -> Memory/1

== system MIL_Test/Test Control/Test Control Architecture/Test Control Conditions/IF Signal@SimStopTime for TC = value1 ==
  Signal : Inport
  Current Sim StopTime : Constant  Value=currentStopTime
  If : If  IfExpression=u1 ~= 1
  Model Info : simulink/Model-Wide Utilities/Model Info  SystemSampleTime=-1  InitialBlockCM=None  BlockCM=None  Frame=on  DisplayStringWithTags=|  HorizontalTextAlignment=Center  LeftAlignmentValue=0.5  SourceBlockDiagram=MIL_Test  TagMaxNumber=20
      | Flag Fullfillment = 1, then condition is true 
      | Flag Fullfillment = 0, then condition is false
  if Signal@t for TC = pass : Subsystem
  "if false, then  TC4 for 200" : Subsystem
  "if true, then  TC2 for 400" : Subsystem
  Fulfillment : Outport
  wires:
  if Signal@t for TC = pass/1(Control Seq1) -> Fulfillment/1
  If/2 -> "if true, then  TC2 for 400"/Action
  If/1 -> "if false, then  TC4 for 200"/Action
  Signal/1 -> if Signal@t for TC = pass/2(Signal1)
  Current Sim StopTime/1 -> if Signal@t for TC = pass/1(@time)

== system MIL_Test/Test Control/Test Control Architecture/Test Control Conditions/IF signal @[timeUp, timeDown] for TC = value1 ==
  Signal : Inport
  TimeDown : Constant  Value=timeDown
  TimeUp : Constant  Value=timeUp
  if Signal@ [TDown,TUp]  for TC = Value : Subsystem
  Fulfillment : Outport
  wires:
  if Signal@ [TDown,TUp]  for TC = Value/1(Control Seq) -> Fulfillment/1
  Signal/1 -> if Signal@ [TDown,TUp]  for TC = Value/3(Signal)
  TimeUp/1 -> if Signal@ [TDown,TUp]  for TC = Value/2(@timeUp)
  TimeDown/1 -> if Signal@ [TDown,TUp]  for TC = Value/1(@timeDown)

== system MIL_Test/Test Control/Test Control Architecture/Test Control Conditions/IF signal@time for TC = value1 ==
  Signal : Inport
  given Time : Constant  Value=time
  if Signal@t for TC = pass : Subsystem
  Fulfillment : Outport
  wires:
  if Signal@t for TC = pass/1(Control Seq) -> Fulfillment/1
  Signal/1 -> if Signal@t for TC = pass/2(Signal1)
  given Time/1 -> if Signal@t for TC = pass/1(@time)

== system MIL_Test/Test Control/Test Control Architecture/Test Control Conditions/IF signal@time1 ==
  Signal : Inport
  Current Sim StopTime : Constant  Value=currentStopTime
  If : If  IfExpression=u1 ~= 1
  Memory : Memory  Orientation=left
  Model Info : simulink/Model-Wide Utilities/Model Info  SystemSampleTime=-1  InitialBlockCM=None  BlockCM=None  Frame=on  DisplayStringWithTags=|  HorizontalTextAlignment=Center  LeftAlignmentValue=0.5  SourceBlockDiagram=MIL_Test  TagMaxNumber=20
      | Flag Fullfillment = 1, then condition is true 
      | Flag Fullfillment = 0, then condition is false
  if Signal@t for TC = pass : Subsystem
  "if false, then  TC4 for 200" : Subsystem
  "if true, then  TC2 for 400" : Subsystem
  Fulfillment : Outport
  wires:
  if Signal@t for TC = pass/1(Control Seq) -> Fulfillment/1
  If/2 -> "if true, then  TC2 for 400"/Action
  If/1 -> "if false, then  TC4 for 200"/Action
  Signal/1 -> if Signal@t for TC = pass/2(Signal1)
  Current Sim StopTime/1 -> if Signal@t for TC = pass/1(@time)

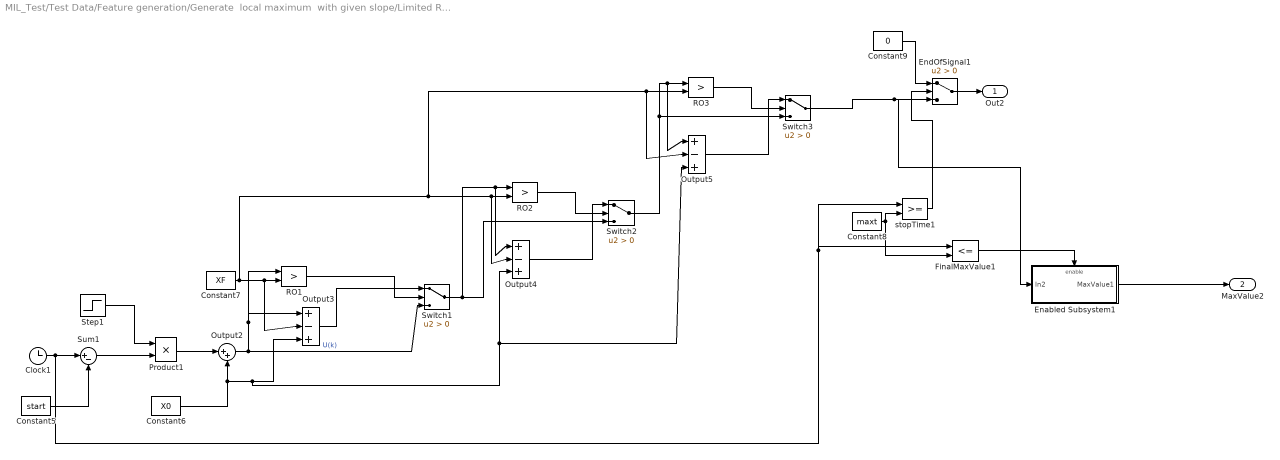
== system MIL_Test/Test Data/Feature generation/Generate  local maximum  with given slope/Limited Ramp Increasing ==
  Clock1 : Clock
      settings: DisableCoverage=on  Decimation=10
  Constant5 : Constant  DisableCoverage=on  Value=start
  Constant6 : Constant  DisableCoverage=on  Value=X0
  Constant7 : Constant  DisableCoverage=on  Value=XF
  Constant8 : Constant  DisableCoverage=on  Value=maxt
  Constant9 : Constant  DisableCoverage=on  Value=0
  Enabled Subsystem1 : Subsystem  TreatAsAtomicUnit=on
  EndOfSignal1 : Switch  Criteria=u2 > Threshold
  FinalMaxValue1 : RelationalOperator  Operator=<=  LogicOutDataTypeMode=Boolean
  Output2 : Sum  Inputs=|++  SaturateOnIntegerOverflow=on  InputSameDT=on
  Output3 : Sum  Inputs=|+-+  SaturateOnIntegerOverflow=on  InputSameDT=on
  Output4 : Sum  Inputs=|+-+  SaturateOnIntegerOverflow=on  InputSameDT=on
  Output5 : Sum  Inputs=|+-+  SaturateOnIntegerOverflow=on  InputSameDT=on
  Product1 : Product  DisableCoverage=on  SaturateOnIntegerOverflow=on  InputSameDT=on
  RO1 : RelationalOperator  Operator=>  LogicOutDataTypeMode=Boolean
  RO2 : RelationalOperator  Operator=>  LogicOutDataTypeMode=Boolean
  RO3 : RelationalOperator  Operator=>  LogicOutDataTypeMode=Boolean
  Step1 : Step  DisableCoverage=on  Time=start  After=slope  SampleTime=0
  Sum1 : Sum  DisableCoverage=on  Inputs=|+-  SaturateOnIntegerOverflow=on  InputSameDT=on
  Switch1 : Switch  Criteria=u2 > Threshold
  Switch2 : Switch  Criteria=u2 > Threshold
  Switch3 : Switch  Criteria=u2 > Threshold
  stopTime1 : RelationalOperator  LogicOutDataTypeMode=Boolean
  Out2 : Outport
  MaxValue2 : Outport  Port=2
  wires:
  Enabled Subsystem1/1(MaxValue1) -> MaxValue2/1
  FinalMaxValue1/1 -> Enabled Subsystem1/Enable
  EndOfSignal1/1 -> Out2/1
  Constant9/1 -> EndOfSignal1/1
  stopTime1/1 -> EndOfSignal1/2
  Constant8/1 -> FinalMaxValue1/2, stopTime1/2
  RO1/1 -> Switch1/2
  Output3/1 -> Switch1/1
  Output2/1 -> Switch1/3, RO1/1, Output3/1  "U(k)"
  Output5/1 -> Switch3/1
  RO3/1 -> Switch3/2
  Switch3/1 -> Enabled Subsystem1/1(In2), EndOfSignal1/3
  Switch2/1 -> Output5/1, RO3/1, Switch3/3
  Output4/1 -> Switch2/1
  RO2/1 -> Switch2/2
  Switch1/1 -> Output4/1, RO2/1, Switch2/3
  Constant7/1 -> Output5/2, RO3/2, Output4/2, RO2/2, Output3/2, RO1/2
  Clock1/1 -> stopTime1/1, FinalMaxValue1/1, Sum1/1
  Constant5/1 -> Sum1/2
  Sum1/1 -> Product1/2
  Constant6/1 -> Output5/3, Output4/3, Output3/3, Output2/2
  Product1/1 -> Output2/1
  Step1/1 -> Product1/1

== system MIL_Test/Test Data/Feature generation/Generate  local maximum  with given slope/Limited Ramp  Decreasing1 ==
  InitialValue : Inport
  Clock : Clock
      settings: DisableCoverage=on  Decimation=10
  Constant : Constant  DisableCoverage=on  Value=maxt
  Constant4 : Constant  DisableCoverage=on  Value=0
  NoStartOfSignal : Switch  Criteria=u2 > Threshold
  NotYetStartTime : RelationalOperator  Operator=<  LogicOutDataTypeMode=Boolean
  Output : Sum  Inputs=|++  SaturateOnIntegerOverflow=on  InputSameDT=on
  Product : Product  DisableCoverage=on  SaturateOnIntegerOverflow=on  InputSameDT=on
  Step : Step  DisableCoverage=on  Time=maxt  After=-slope  SampleTime=0
  Sum : Sum  DisableCoverage=on  Inputs=|+-  SaturateOnIntegerOverflow=on  InputSameDT=on
  Out1 : Outport
  wires:
  NoStartOfSignal/1 -> Out1/1
  Constant4/1 -> NoStartOfSignal/1
  NotYetStartTime/1 -> NoStartOfSignal/2
  Step/1 -> Product/1
  Product/1 -> Output/1
  InitialValue/1 -> Output/2
  Output/1 -> NoStartOfSignal/3
  Sum/1 -> Product/2
  Constant/1 -> NotYetStartTime/2, Sum/2
  Clock/1 -> NotYetStartTime/1, Sum/1

== system MIL_Test/Test Data/Feature generation/Generate complete step/Hold Time ==
  Clock : Inport
  Enable : EnablePort
  Write : DataStoreWrite  DataStoreName=triggerTime  SampleTime=-1
  wires:
  Clock/1 -> Write/1

== system MIL_Test/Test Data/Feature generation/Generate complete step/Hold Value ==
  In1 : Inport
  Enable : EnablePort
  v_Des : Outport
  wires:
  In1/1 -> v_Des/1

== system MIL_Test/Test Data/Test Data Architecture/<Test data generator>/<Requirement name> ==
  Out Bus : Inport
  <Preconditions name> : Subsystem
  Initialisation & Stabilisation : Subsystem
  Sequencing of test data in time due to Preconditions : Stateflow chart
  switch <signal1> : MultiPortSwitch  Inputs=2
  <signal1> : Outport
  wires:
  Initialisation & Stabilisation/1(<signal1>) -> switch <signal1>/3
  <Preconditions name>/2(<signal1>) -> switch <signal1>/2
  Sequencing of test data in time due to Preconditions/1(TDPre) -> switch <signal1>/1
  <Preconditions name>/1(Activate) -> Sequencing of test data in time due to Preconditions/1(Activate)
  switch <signal1>/1 -> <signal1>/1
  Out Bus/1 -> <Preconditions name>/1(Out Bus)
